simulink model "GolfSwingZVCF"  (R2024a)
settings: Solver=VariableStepAuto  StartTime=0.0  StopTime=StopTime  MaxStep=0.001  RelTol=1e-3
PreLoadFcn:
  | cd(matlabdrive);
PostLoadFcn:
  | %run SCRIPT_mdlWksGenerate.m;
  | mdlWks=get_param('GolfSwingZVCF','ModelWorkspace');
  | mdlWks.DataSource = 'MAT-File';
  | mdlWks.FileName = 'ModelInputs.mat';
  | mdlWks.reload;
model workspace: external: MAT-File ModelInputsZVCF.mat (data not in the file)
undefined symbols (not defined in the file): JointTorqueHip, JointTorqueLElbow, JointTorqueLScap, JointTorqueLShoulder, JointTorqueLWrist, JointTorqueRElbow, JointTorqueRScap, JointTorqueRShoulder, JointTorqueRWrist, JointTorqueTorso, X, Y, Z
libraries: nesl_utility x286, sm_lib x176, matrix_library x11, simulink_extras x2
(part 9 of 9)

== system GolfSwingZVCF/Club/Revolute Joint Shaft Models/12 Segment Shaft (1 Degree Prestress)/ShaftPhysicalConfig/Subsystem8 ==
  Kill : Inport
  KDamp9 : Inport  Port=2
  KShaft9 : Inport  Port=3
  Add : Sum
  Invert : Constant  Value=-1
  Invert1 : Constant  Value=-1
  PS-Simulink Converter11 : nesl_utility/PS-Simulink Converter  PhysicalDomain=network_engine_domain  SubClassName=ps_output  LeftPortType=input  RightPortType=output  PseudoPeriodic=off  Frequencies=[]  VectorFormat=1-D array  Unit=inherit  AffineConversion=off
  PS-Simulink Converter16 : nesl_utility/PS-Simulink Converter  PhysicalDomain=network_engine_domain  SubClassName=ps_output  LeftPortType=input  RightPortType=output  PseudoPeriodic=off  Frequencies=[]  VectorFormat=inherit  Unit=inherit  AffineConversion=off
  Product : Product  Inputs=3
  Product2 : Product
  Product3 : Product  Inputs=3
  Simulink-PS Converter : nesl_utility/Simulink-PS Converter  PhysicalDomain=network_engine_domain  SubClassName=ps_input  LeftPortType=input  RightPortType=output  PseudoPeriodic=off  Frequencies=[]  NoiseDistribution=none  NoiseParameters=[]  Unit=1  AffineConversion=off  FilteringAndDerivatives=provide  SimscapeFilterOrder=1  InputFilterTimeConstant=0.001  UdotUserProvided=0
  Torque9 : PMIOPort  Side=Right
  AV9 : PMIOPort  Port=2  Side=Right
  Position9 : PMIOPort  Port=3  Side=Right
  wires:
  Product3/1 -> Add/1
  Kill/1 -> Product2/1
  KShaft9/1 -> Product/2
  Invert/1 -> Product/3
  Invert1/1 -> Product3/3
  Product/1 -> Add/2
  KDamp9/1 -> Product3/2
  Product2/1 -> Simulink-PS Converter/1
  Add/1 -> Product2/2
  PS-Simulink Converter11/1 -> Product/1
  PS-Simulink Converter16/1 -> Product3/1
  connections:
  Simulink-PS Converter/RConn1 -- Torque9/RConn1
  AV9/RConn1 -- PS-Simulink Converter16/LConn1
  PS-Simulink Converter11/LConn1 -- Position9/RConn1

== system GolfSwingZVCF/Club/Revolute Joint Shaft Models/12 Segment Shaft (1 Degree Prestress)/ShaftPhysicalConfig/Subsystem9 ==
  Kill : Inport
  KDamp10 : Inport  Port=2
  KShaft10 : Inport  Port=3
  Add : Sum
  Invert : Constant  Value=-1
  Invert1 : Constant  Value=-1
  PS-Simulink Converter11 : nesl_utility/PS-Simulink Converter  PhysicalDomain=network_engine_domain  SubClassName=ps_output  LeftPortType=input  RightPortType=output  PseudoPeriodic=off  Frequencies=[]  VectorFormat=1-D array  Unit=inherit  AffineConversion=off
  PS-Simulink Converter16 : nesl_utility/PS-Simulink Converter  PhysicalDomain=network_engine_domain  SubClassName=ps_output  LeftPortType=input  RightPortType=output  PseudoPeriodic=off  Frequencies=[]  VectorFormat=inherit  Unit=inherit  AffineConversion=off
  Product : Product  Inputs=3
  Product2 : Product
  Product3 : Product  Inputs=3
  Simulink-PS Converter : nesl_utility/Simulink-PS Converter  PhysicalDomain=network_engine_domain  SubClassName=ps_input  LeftPortType=input  RightPortType=output  PseudoPeriodic=off  Frequencies=[]  NoiseDistribution=none  NoiseParameters=[]  Unit=1  AffineConversion=off  FilteringAndDerivatives=provide  SimscapeFilterOrder=1  InputFilterTimeConstant=0.001  UdotUserProvided=0
  Torque10 : PMIOPort  Side=Right
  AV10 : PMIOPort  Port=2  Side=Right
  Position10 : PMIOPort  Port=3  Side=Right
  wires:
  Product3/1 -> Add/1
  Kill/1 -> Product2/1
  Invert/1 -> Product/3
  PS-Simulink Converter16/1 -> Product3/1
  Invert1/1 -> Product3/3
  Product/1 -> Add/2
  KDamp10/1 -> Product3/2
  Product2/1 -> Simulink-PS Converter/1
  Add/1 -> Product2/2
  PS-Simulink Converter11/1 -> Product/1
  KShaft10/1 -> Product/2
  connections:
  AV10/RConn1 -- PS-Simulink Converter16/LConn1
  Simulink-PS Converter/RConn1 -- Torque10/RConn1
  PS-Simulink Converter11/LConn1 -- Position10/RConn1

== system GolfSwingZVCF/Club/Revolute Joint Shaft Models/12 Segment Shaft (No Prestress) /ShaftPhysicalConfig/Subsystem ==
  Kill : Inport
  KDamp1 : Inport  Port=2
  KShaft1 : Inport  Port=3
  Add : Sum
  Invert : Constant  Value=-1
  Invert1 : Constant  Value=-1
  PS-Simulink Converter11 : nesl_utility/PS-Simulink Converter  PhysicalDomain=network_engine_domain  SubClassName=ps_output  LeftPortType=input  RightPortType=output  PseudoPeriodic=off  Frequencies=[]  VectorFormat=1-D array  Unit=inherit  AffineConversion=off
  PS-Simulink Converter16 : nesl_utility/PS-Simulink Converter  PhysicalDomain=network_engine_domain  SubClassName=ps_output  LeftPortType=input  RightPortType=output  PseudoPeriodic=off  Frequencies=[]  VectorFormat=inherit  Unit=inherit  AffineConversion=off
  Product : Product  Inputs=3
  Product2 : Product
  Product3 : Product  Inputs=3
  Simulink-PS Converter : nesl_utility/Simulink-PS Converter  PhysicalDomain=network_engine_domain  SubClassName=ps_input  LeftPortType=input  RightPortType=output  PseudoPeriodic=off  Frequencies=[]  NoiseDistribution=none  NoiseParameters=[]  Unit=1  AffineConversion=off  FilteringAndDerivatives=provide  SimscapeFilterOrder=1  InputFilterTimeConstant=0.001  UdotUserProvided=0
  Torque1 : PMIOPort  Side=Right
  AV1 : PMIOPort  Port=2  Side=Right
  Position1 : PMIOPort  Port=3  Side=Right
  wires:
  Product3/1 -> Add/1
  Kill/1 -> Product2/1
  KShaft1/1 -> Product/2
  Invert/1 -> Product/3
  PS-Simulink Converter16/1 -> Product3/1
  Invert1/1 -> Product3/3
  Product/1 -> Add/2
  KDamp1/1 -> Product3/2
  Product2/1 -> Simulink-PS Converter/1
  Add/1 -> Product2/2
  PS-Simulink Converter11/1 -> Product/1
  connections:
  AV1/RConn1 -- PS-Simulink Converter16/LConn1
  Simulink-PS Converter/RConn1 -- Torque1/RConn1
  PS-Simulink Converter11/LConn1 -- Position1/RConn1

== system GolfSwingZVCF/Club/Revolute Joint Shaft Models/12 Segment Shaft (No Prestress) /ShaftPhysicalConfig/Subsystem1 ==
  Kill : Inport
  KDamp2 : Inport  Port=2
  KShaft2 : Inport  Port=3
  Add : Sum
  Invert : Constant  Value=-1
  Invert1 : Constant  Value=-1
  PS-Simulink Converter11 : nesl_utility/PS-Simulink Converter  PhysicalDomain=network_engine_domain  SubClassName=ps_output  LeftPortType=input  RightPortType=output  PseudoPeriodic=off  Frequencies=[]  VectorFormat=1-D array  Unit=inherit  AffineConversion=off
  PS-Simulink Converter16 : nesl_utility/PS-Simulink Converter  PhysicalDomain=network_engine_domain  SubClassName=ps_output  LeftPortType=input  RightPortType=output  PseudoPeriodic=off  Frequencies=[]  VectorFormat=inherit  Unit=inherit  AffineConversion=off
  Product : Product  Inputs=3
  Product2 : Product
  Product3 : Product  Inputs=3
  Simulink-PS Converter : nesl_utility/Simulink-PS Converter  PhysicalDomain=network_engine_domain  SubClassName=ps_input  LeftPortType=input  RightPortType=output  PseudoPeriodic=off  Frequencies=[]  NoiseDistribution=none  NoiseParameters=[]  Unit=1  AffineConversion=off  FilteringAndDerivatives=provide  SimscapeFilterOrder=1  InputFilterTimeConstant=0.001  UdotUserProvided=0
  Torque2 : PMIOPort  Side=Right
  AV2 : PMIOPort  Port=2  Side=Right
  Position2 : PMIOPort  Port=3  Side=Right
  wires:
  Product3/1 -> Add/1
  Kill/1 -> Product2/1
  Invert/1 -> Product/3
  PS-Simulink Converter16/1 -> Product3/1
  Invert1/1 -> Product3/3
  Product/1 -> Add/2
  Product2/1 -> Simulink-PS Converter/1
  Add/1 -> Product2/2
  PS-Simulink Converter11/1 -> Product/1
  KDamp2/1 -> Product3/2
  KShaft2/1 -> Product/2
  connections:
  AV2/RConn1 -- PS-Simulink Converter16/LConn1
  Simulink-PS Converter/RConn1 -- Torque2/RConn1
  PS-Simulink Converter11/LConn1 -- Position2/RConn1

== system GolfSwingZVCF/Club/Revolute Joint Shaft Models/12 Segment Shaft (No Prestress) /ShaftPhysicalConfig/Subsystem10 ==
  Kill : Inport
  KDamp11 : Inport  Port=2
  KShaft11 : Inport  Port=3
  Add : Sum
  Invert : Constant  Value=-1
  Invert1 : Constant  Value=-1
  PS-Simulink Converter11 : nesl_utility/PS-Simulink Converter  PhysicalDomain=network_engine_domain  SubClassName=ps_output  LeftPortType=input  RightPortType=output  PseudoPeriodic=off  Frequencies=[]  VectorFormat=1-D array  Unit=inherit  AffineConversion=off
  PS-Simulink Converter16 : nesl_utility/PS-Simulink Converter  PhysicalDomain=network_engine_domain  SubClassName=ps_output  LeftPortType=input  RightPortType=output  PseudoPeriodic=off  Frequencies=[]  VectorFormat=inherit  Unit=inherit  AffineConversion=off
  Product : Product  Inputs=3
  Product2 : Product
  Product3 : Product  Inputs=3
  Simulink-PS Converter : nesl_utility/Simulink-PS Converter  PhysicalDomain=network_engine_domain  SubClassName=ps_input  LeftPortType=input  RightPortType=output  PseudoPeriodic=off  Frequencies=[]  NoiseDistribution=none  NoiseParameters=[]  Unit=1  AffineConversion=off  FilteringAndDerivatives=provide  SimscapeFilterOrder=1  InputFilterTimeConstant=0.001  UdotUserProvided=0
  Torque11 : PMIOPort  Side=Right
  AV11 : PMIOPort  Port=2  Side=Right
  Position11 : PMIOPort  Port=3  Side=Right
  wires:
  Product3/1 -> Add/1
  Kill/1 -> Product2/1
  Invert/1 -> Product/3
  PS-Simulink Converter16/1 -> Product3/1
  Invert1/1 -> Product3/3
  Product/1 -> Add/2
  Product2/1 -> Simulink-PS Converter/1
  Add/1 -> Product2/2
  PS-Simulink Converter11/1 -> Product/1
  KDamp11/1 -> Product3/2
  KShaft11/1 -> Product/2
  connections:
  AV11/RConn1 -- PS-Simulink Converter16/LConn1
  Simulink-PS Converter/RConn1 -- Torque11/RConn1
  PS-Simulink Converter11/LConn1 -- Position11/RConn1

== system GolfSwingZVCF/Club/Revolute Joint Shaft Models/12 Segment Shaft (No Prestress) /ShaftPhysicalConfig/Subsystem2 ==
  Kill : Inport
  KDamp3 : Inport  Port=2
  KShaft3 : Inport  Port=3
  Add : Sum
  Invert : Constant  Value=-1
  Invert1 : Constant  Value=-1
  PS-Simulink Converter11 : nesl_utility/PS-Simulink Converter  PhysicalDomain=network_engine_domain  SubClassName=ps_output  LeftPortType=input  RightPortType=output  PseudoPeriodic=off  Frequencies=[]  VectorFormat=1-D array  Unit=inherit  AffineConversion=off
  PS-Simulink Converter16 : nesl_utility/PS-Simulink Converter  PhysicalDomain=network_engine_domain  SubClassName=ps_output  LeftPortType=input  RightPortType=output  PseudoPeriodic=off  Frequencies=[]  VectorFormat=inherit  Unit=inherit  AffineConversion=off
  Product : Product  Inputs=3
  Product2 : Product
  Product3 : Product  Inputs=3
  Simulink-PS Converter : nesl_utility/Simulink-PS Converter  PhysicalDomain=network_engine_domain  SubClassName=ps_input  LeftPortType=input  RightPortType=output  PseudoPeriodic=off  Frequencies=[]  NoiseDistribution=none  NoiseParameters=[]  Unit=1  AffineConversion=off  FilteringAndDerivatives=provide  SimscapeFilterOrder=1  InputFilterTimeConstant=0.001  UdotUserProvided=0
  Torque3 : PMIOPort  Side=Right
  AV3 : PMIOPort  Port=2  Side=Right
  Position3 : PMIOPort  Port=3  Side=Right
  wires:
  Product3/1 -> Add/1
  Kill/1 -> Product2/1
  KShaft3/1 -> Product/2
  Invert/1 -> Product/3
  PS-Simulink Converter16/1 -> Product3/1
  Invert1/1 -> Product3/3
  Product/1 -> Add/2
  KDamp3/1 -> Product3/2
  Product2/1 -> Simulink-PS Converter/1
  Add/1 -> Product2/2
  PS-Simulink Converter11/1 -> Product/1
  connections:
  AV3/RConn1 -- PS-Simulink Converter16/LConn1
  Simulink-PS Converter/RConn1 -- Torque3/RConn1
  PS-Simulink Converter11/LConn1 -- Position3/RConn1

== system GolfSwingZVCF/Club/Revolute Joint Shaft Models/12 Segment Shaft (No Prestress) /ShaftPhysicalConfig/Subsystem3 ==
  Kill : Inport
  KDamp4 : Inport  Port=2
  KShaft4 : Inport  Port=3
  Add : Sum
  Invert : Constant  Value=-1
  Invert1 : Constant  Value=-1
  PS-Simulink Converter11 : nesl_utility/PS-Simulink Converter  PhysicalDomain=network_engine_domain  SubClassName=ps_output  LeftPortType=input  RightPortType=output  PseudoPeriodic=off  Frequencies=[]  VectorFormat=1-D array  Unit=inherit  AffineConversion=off
  PS-Simulink Converter16 : nesl_utility/PS-Simulink Converter  PhysicalDomain=network_engine_domain  SubClassName=ps_output  LeftPortType=input  RightPortType=output  PseudoPeriodic=off  Frequencies=[]  VectorFormat=inherit  Unit=inherit  AffineConversion=off
  Product : Product  Inputs=3
  Product2 : Product
  Product3 : Product  Inputs=3
  Simulink-PS Converter : nesl_utility/Simulink-PS Converter  PhysicalDomain=network_engine_domain  SubClassName=ps_input  LeftPortType=input  RightPortType=output  PseudoPeriodic=off  Frequencies=[]  NoiseDistribution=none  NoiseParameters=[]  Unit=1  AffineConversion=off  FilteringAndDerivatives=provide  SimscapeFilterOrder=1  InputFilterTimeConstant=0.001  UdotUserProvided=0
  Torque4 : PMIOPort  Side=Right
  AV4 : PMIOPort  Port=2  Side=Right
  Position4 : PMIOPort  Port=3  Side=Right
  wires:
  Product3/1 -> Add/1
  KShaft4/1 -> Product/2
  Invert/1 -> Product/3
  PS-Simulink Converter16/1 -> Product3/1
  Invert1/1 -> Product3/3
  Product/1 -> Add/2
  KDamp4/1 -> Product3/2
  Product2/1 -> Simulink-PS Converter/1
  Add/1 -> Product2/2
  PS-Simulink Converter11/1 -> Product/1
  Kill/1 -> Product2/1
  connections:
  AV4/RConn1 -- PS-Simulink Converter16/LConn1
  Simulink-PS Converter/RConn1 -- Torque4/RConn1
  PS-Simulink Converter11/LConn1 -- Position4/RConn1

== system GolfSwingZVCF/Club/Revolute Joint Shaft Models/12 Segment Shaft (No Prestress) /ShaftPhysicalConfig/Subsystem4 ==
  Kill : Inport
  KDamp5 : Inport  Port=2
  KShaft5 : Inport  Port=3
  Add : Sum
  Invert : Constant  Value=-1
  Invert1 : Constant  Value=-1
  PS-Simulink Converter11 : nesl_utility/PS-Simulink Converter  PhysicalDomain=network_engine_domain  SubClassName=ps_output  LeftPortType=input  RightPortType=output  PseudoPeriodic=off  Frequencies=[]  VectorFormat=1-D array  Unit=inherit  AffineConversion=off
  PS-Simulink Converter16 : nesl_utility/PS-Simulink Converter  PhysicalDomain=network_engine_domain  SubClassName=ps_output  LeftPortType=input  RightPortType=output  PseudoPeriodic=off  Frequencies=[]  VectorFormat=inherit  Unit=inherit  AffineConversion=off
  Product : Product  Inputs=3
  Product2 : Product
  Product3 : Product  Inputs=3
  Simulink-PS Converter : nesl_utility/Simulink-PS Converter  PhysicalDomain=network_engine_domain  SubClassName=ps_input  LeftPortType=input  RightPortType=output  PseudoPeriodic=off  Frequencies=[]  NoiseDistribution=none  NoiseParameters=[]  Unit=1  AffineConversion=off  FilteringAndDerivatives=provide  SimscapeFilterOrder=1  InputFilterTimeConstant=0.001  UdotUserProvided=0
  Torque5 : PMIOPort  Side=Right
  AV2 : PMIOPort  Port=2  Side=Right
  Position5 : PMIOPort  Port=3  Side=Right
  wires:
  Product3/1 -> Add/1
  KShaft5/1 -> Product/2
  Invert/1 -> Product/3
  PS-Simulink Converter16/1 -> Product3/1
  Invert1/1 -> Product3/3
  Product/1 -> Add/2
  KDamp5/1 -> Product3/2
  Product2/1 -> Simulink-PS Converter/1
  Add/1 -> Product2/2
  PS-Simulink Converter11/1 -> Product/1
  Kill/1 -> Product2/1
  connections:
  AV2/RConn1 -- PS-Simulink Converter16/LConn1
  Simulink-PS Converter/RConn1 -- Torque5/RConn1
  PS-Simulink Converter11/LConn1 -- Position5/RConn1

== system GolfSwingZVCF/Club/Revolute Joint Shaft Models/12 Segment Shaft (No Prestress) /ShaftPhysicalConfig/Subsystem5 ==
  Kill : Inport
  KDamp6 : Inport  Port=2
  KShaft6 : Inport  Port=3
  Add : Sum
  Invert : Constant  Value=-1
  Invert1 : Constant  Value=-1
  PS-Simulink Converter11 : nesl_utility/PS-Simulink Converter  PhysicalDomain=network_engine_domain  SubClassName=ps_output  LeftPortType=input  RightPortType=output  PseudoPeriodic=off  Frequencies=[]  VectorFormat=1-D array  Unit=inherit  AffineConversion=off
  PS-Simulink Converter16 : nesl_utility/PS-Simulink Converter  PhysicalDomain=network_engine_domain  SubClassName=ps_output  LeftPortType=input  RightPortType=output  PseudoPeriodic=off  Frequencies=[]  VectorFormat=inherit  Unit=inherit  AffineConversion=off
  Product : Product  Inputs=3
  Product2 : Product
  Product3 : Product  Inputs=3
  Simulink-PS Converter : nesl_utility/Simulink-PS Converter  PhysicalDomain=network_engine_domain  SubClassName=ps_input  LeftPortType=input  RightPortType=output  PseudoPeriodic=off  Frequencies=[]  NoiseDistribution=none  NoiseParameters=[]  Unit=1  AffineConversion=off  FilteringAndDerivatives=provide  SimscapeFilterOrder=1  InputFilterTimeConstant=0.001  UdotUserProvided=0
  Torque6 : PMIOPort  Side=Right
  AV6 : PMIOPort  Port=2  Side=Right
  Position6 : PMIOPort  Port=3  Side=Right
  wires:
  Product3/1 -> Add/1
  Kill/1 -> Product2/1
  KShaft6/1 -> Product/2
  Invert/1 -> Product/3
  PS-Simulink Converter16/1 -> Product3/1
  Invert1/1 -> Product3/3
  Product/1 -> Add/2
  KDamp6/1 -> Product3/2
  Product2/1 -> Simulink-PS Converter/1
  Add/1 -> Product2/2
  PS-Simulink Converter11/1 -> Product/1
  connections:
  AV6/RConn1 -- PS-Simulink Converter16/LConn1
  Simulink-PS Converter/RConn1 -- Torque6/RConn1
  PS-Simulink Converter11/LConn1 -- Position6/RConn1

== system GolfSwingZVCF/Club/Revolute Joint Shaft Models/12 Segment Shaft (No Prestress) /ShaftPhysicalConfig/Subsystem6 ==
  Kill : Inport
  KDamp7 : Inport  Port=2
  KShaft7 : Inport  Port=3
  Add : Sum
  Invert : Constant  Value=-1
  Invert1 : Constant  Value=-1
  PS-Simulink Converter11 : nesl_utility/PS-Simulink Converter  PhysicalDomain=network_engine_domain  SubClassName=ps_output  LeftPortType=input  RightPortType=output  PseudoPeriodic=off  Frequencies=[]  VectorFormat=1-D array  Unit=inherit  AffineConversion=off
  PS-Simulink Converter16 : nesl_utility/PS-Simulink Converter  PhysicalDomain=network_engine_domain  SubClassName=ps_output  LeftPortType=input  RightPortType=output  PseudoPeriodic=off  Frequencies=[]  VectorFormat=inherit  Unit=inherit  AffineConversion=off
  Product : Product  Inputs=3
  Product2 : Product
  Product3 : Product  Inputs=3
  Simulink-PS Converter : nesl_utility/Simulink-PS Converter  PhysicalDomain=network_engine_domain  SubClassName=ps_input  LeftPortType=input  RightPortType=output  PseudoPeriodic=off  Frequencies=[]  NoiseDistribution=none  NoiseParameters=[]  Unit=1  AffineConversion=off  FilteringAndDerivatives=provide  SimscapeFilterOrder=1  InputFilterTimeConstant=0.001  UdotUserProvided=0
  Torque7 : PMIOPort  Side=Right
  AV7 : PMIOPort  Port=2  Side=Right
  Position7 : PMIOPort  Port=3  Side=Right
  wires:
  Product3/1 -> Add/1
  Kill/1 -> Product2/1
  KShaft7/1 -> Product/2
  Invert/1 -> Product/3
  PS-Simulink Converter16/1 -> Product3/1
  Invert1/1 -> Product3/3
  Product/1 -> Add/2
  KDamp7/1 -> Product3/2
  Product2/1 -> Simulink-PS Converter/1
  Add/1 -> Product2/2
  PS-Simulink Converter11/1 -> Product/1
  connections:
  AV7/RConn1 -- PS-Simulink Converter16/LConn1
  Simulink-PS Converter/RConn1 -- Torque7/RConn1
  PS-Simulink Converter11/LConn1 -- Position7/RConn1

== system GolfSwingZVCF/Club/Revolute Joint Shaft Models/12 Segment Shaft (No Prestress) /ShaftPhysicalConfig/Subsystem7 ==
  Kill : Inport
  KDamp8 : Inport  Port=2
  KShaft8 : Inport  Port=3
  Add : Sum
  Invert : Constant  Value=-1
  Invert1 : Constant  Value=-1
  PS-Simulink Converter11 : nesl_utility/PS-Simulink Converter  PhysicalDomain=network_engine_domain  SubClassName=ps_output  LeftPortType=input  RightPortType=output  PseudoPeriodic=off  Frequencies=[]  VectorFormat=1-D array  Unit=inherit  AffineConversion=off
  PS-Simulink Converter16 : nesl_utility/PS-Simulink Converter  PhysicalDomain=network_engine_domain  SubClassName=ps_output  LeftPortType=input  RightPortType=output  PseudoPeriodic=off  Frequencies=[]  VectorFormat=inherit  Unit=inherit  AffineConversion=off
  Product : Product  Inputs=3
  Product2 : Product
  Product3 : Product  Inputs=3
  Simulink-PS Converter : nesl_utility/Simulink-PS Converter  PhysicalDomain=network_engine_domain  SubClassName=ps_input  LeftPortType=input  RightPortType=output  PseudoPeriodic=off  Frequencies=[]  NoiseDistribution=none  NoiseParameters=[]  Unit=1  AffineConversion=off  FilteringAndDerivatives=provide  SimscapeFilterOrder=1  InputFilterTimeConstant=0.001  UdotUserProvided=0
  Torque8 : PMIOPort  Side=Right
  AV8 : PMIOPort  Port=2  Side=Right
  Position8 : PMIOPort  Port=3  Side=Right
  wires:
  Product3/1 -> Add/1
  Kill/1 -> Product2/1
  KShaft8/1 -> Product/2
  Invert/1 -> Product/3
  PS-Simulink Converter16/1 -> Product3/1
  Invert1/1 -> Product3/3
  Product/1 -> Add/2
  Product2/1 -> Simulink-PS Converter/1
  Add/1 -> Product2/2
  PS-Simulink Converter11/1 -> Product/1
  KDamp8/1 -> Product3/2
  connections:
  AV8/RConn1 -- PS-Simulink Converter16/LConn1
  Simulink-PS Converter/RConn1 -- Torque8/RConn1
  PS-Simulink Converter11/LConn1 -- Position8/RConn1

== system GolfSwingZVCF/Club/Revolute Joint Shaft Models/12 Segment Shaft (No Prestress) /ShaftPhysicalConfig/Subsystem8 ==
  Kill : Inport
  KDamp9 : Inport  Port=2
  KShaft9 : Inport  Port=3
  Add : Sum
  Invert : Constant  Value=-1
  Invert1 : Constant  Value=-1
  PS-Simulink Converter11 : nesl_utility/PS-Simulink Converter  PhysicalDomain=network_engine_domain  SubClassName=ps_output  LeftPortType=input  RightPortType=output  PseudoPeriodic=off  Frequencies=[]  VectorFormat=1-D array  Unit=inherit  AffineConversion=off
  PS-Simulink Converter16 : nesl_utility/PS-Simulink Converter  PhysicalDomain=network_engine_domain  SubClassName=ps_output  LeftPortType=input  RightPortType=output  PseudoPeriodic=off  Frequencies=[]  VectorFormat=inherit  Unit=inherit  AffineConversion=off
  Product : Product  Inputs=3
  Product2 : Product
  Product3 : Product  Inputs=3
  Simulink-PS Converter : nesl_utility/Simulink-PS Converter  PhysicalDomain=network_engine_domain  SubClassName=ps_input  LeftPortType=input  RightPortType=output  PseudoPeriodic=off  Frequencies=[]  NoiseDistribution=none  NoiseParameters=[]  Unit=1  AffineConversion=off  FilteringAndDerivatives=provide  SimscapeFilterOrder=1  InputFilterTimeConstant=0.001  UdotUserProvided=0
  Torque9 : PMIOPort  Side=Right
  AV9 : PMIOPort  Port=2  Side=Right
  Position9 : PMIOPort  Port=3  Side=Right
  wires:
  Product3/1 -> Add/1
  Kill/1 -> Product2/1
  KShaft9/1 -> Product/2
  Invert/1 -> Product/3
  Invert1/1 -> Product3/3
  Product/1 -> Add/2
  KDamp9/1 -> Product3/2
  Product2/1 -> Simulink-PS Converter/1
  Add/1 -> Product2/2
  PS-Simulink Converter11/1 -> Product/1
  PS-Simulink Converter16/1 -> Product3/1
  connections:
  Simulink-PS Converter/RConn1 -- Torque9/RConn1
  AV9/RConn1 -- PS-Simulink Converter16/LConn1
  PS-Simulink Converter11/LConn1 -- Position9/RConn1

== system GolfSwingZVCF/Club/Revolute Joint Shaft Models/12 Segment Shaft (No Prestress) /ShaftPhysicalConfig/Subsystem9 ==
  Kill : Inport
  KDamp10 : Inport  Port=2
  KShaft10 : Inport  Port=3
  Add : Sum
  Invert : Constant  Value=-1
  Invert1 : Constant  Value=-1
  PS-Simulink Converter11 : nesl_utility/PS-Simulink Converter  PhysicalDomain=network_engine_domain  SubClassName=ps_output  LeftPortType=input  RightPortType=output  PseudoPeriodic=off  Frequencies=[]  VectorFormat=1-D array  Unit=inherit  AffineConversion=off
  PS-Simulink Converter16 : nesl_utility/PS-Simulink Converter  PhysicalDomain=network_engine_domain  SubClassName=ps_output  LeftPortType=input  RightPortType=output  PseudoPeriodic=off  Frequencies=[]  VectorFormat=inherit  Unit=inherit  AffineConversion=off
  Product : Product  Inputs=3
  Product2 : Product
  Product3 : Product  Inputs=3
  Simulink-PS Converter : nesl_utility/Simulink-PS Converter  PhysicalDomain=network_engine_domain  SubClassName=ps_input  LeftPortType=input  RightPortType=output  PseudoPeriodic=off  Frequencies=[]  NoiseDistribution=none  NoiseParameters=[]  Unit=1  AffineConversion=off  FilteringAndDerivatives=provide  SimscapeFilterOrder=1  InputFilterTimeConstant=0.001  UdotUserProvided=0
  Torque10 : PMIOPort  Side=Right
  AV10 : PMIOPort  Port=2  Side=Right
  Position10 : PMIOPort  Port=3  Side=Right
  wires:
  Product3/1 -> Add/1
  Kill/1 -> Product2/1
  Invert/1 -> Product/3
  PS-Simulink Converter16/1 -> Product3/1
  Invert1/1 -> Product3/3
  Product/1 -> Add/2
  KDamp10/1 -> Product3/2
  Product2/1 -> Simulink-PS Converter/1
  Add/1 -> Product2/2
  PS-Simulink Converter11/1 -> Product/1
  KShaft10/1 -> Product/2
  connections:
  AV10/RConn1 -- PS-Simulink Converter16/LConn1
  Simulink-PS Converter/RConn1 -- Torque10/RConn1
  PS-Simulink Converter11/LConn1 -- Position10/RConn1

== matlab function GolfSwingZVCF/Club/Impact Model/Golf Ball Reaction Force ==
  data: u input; FImpact output
function FImpact = fcn(u)

FImpact=-u*1.5*.44704*.0459/.0005;
%Impact Time = 0.0005 s
%Golf Ball Mass = 0.0459 g
%MPH to m/s conversion = 0.44704 m/s / MPH
%Smash Factor = 1.5

== matlab function GolfSwingZVCF/Club/Clubhead Air Resistance Calculator/Drag Function ==
  data: u input; FDrag output
function FDrag = fcn(u)

FDrag = -1/2*1.225*3.1415927*(2.5/39)^2*0.47*u^2;
%Shape Factor = 0.47
%Air Density = 1.225 kg/m3
%CH Radius = 2.5"
%Fd=-1/2*Density*ShapeFactor*CSA*v^2

== matlab function GolfSwingZVCF/RJM Inputs/Hip Input Torque ==
  data: JointTorqueHipsInput input; JointTorqueHips output
function JointTorqueHips = fcn(JointTorqueHipsInput)
JointTorqueHips=JointTorqueHipsInput;

== matlab function GolfSwingZVCF/RJM Inputs/Torso Input Torque ==
  data: JointTorqueTorsoInput input; JointTorqueHips output
function JointTorqueHips = fcn(JointTorqueTorsoInput)
JointTorqueHips=JointTorqueTorsoInput;

== matlab function GolfSwingZVCF/RJM Inputs/LScap Input Torque ==
  data: JointTorqueHipsInput input; JointTorqueHips output
function JointTorqueHips = fcn(JointTorqueHipsInput)
JointTorqueHips=JointTorqueHipsInput;

== matlab function GolfSwingZVCF/RJM Inputs/RScap Input Torque ==
  data: JointTorqueRScapInput input; JointTorqueRScap output
function JointTorqueRScap = fcn(JointTorqueRScapInput)
JointTorqueRScap=JointTorqueRScapInput;

== matlab function GolfSwingZVCF/RJM Inputs/LShoulder Input Torque ==
  data: JointTorqueLShoulderInput input; JointTorqueLShoulder output
function JointTorqueLShoulder = fcn(JointTorqueLShoulderInput)
JointTorqueLShoulder=JointTorqueLShoulderInput;

== matlab function GolfSwingZVCF/RJM Inputs/LWrist Input Torque ==
  data: JointTorqueLWristInput input; JointTorqueLWrist output
function JointTorqueLWrist = fcn(JointTorqueLWristInput)
JointTorqueLWrist=JointTorqueLWristInput;

== matlab function GolfSwingZVCF/RJM Inputs/RShoulder Input Torque ==
  data: JointTorqueRShoulderInput input; JointTorqueRShoulder output
function JointTorqueRShoulder = fcn(JointTorqueRShoulderInput)
JointTorqueRShoulder=JointTorqueRShoulderInput;

== matlab function GolfSwingZVCF/RJM Inputs/RWrist Input Torque ==
  data: JointTorqueRWristInput input; JointTorqueRWrist output
function JointTorqueRWrist = fcn(JointTorqueRWristInput)
JointTorqueRWrist=JointTorqueRWristInput;

== matlab function GolfSwingZVCF/RJM Inputs/Left Elbow Input Torque ==
  data: JointTorqueLElbowInput input; JointTorqueLElbow output
function JointTorqueLElbow = fcn(JointTorqueLElbowInput)
JointTorqueLElbow=JointTorqueLElbowInput;

== matlab function GolfSwingZVCF/RJM Inputs/Right Elbow Input Torque ==
  data: JointTorqueRElbowInput input; JointTorqueRElbow output
function JointTorqueRElbow = fcn(JointTorqueRElbowInput)
JointTorqueRElbow=JointTorqueRElbowInput;

== matlab function GolfSwingZVCF/Club/CHGlobal/Filtering Block/MATLAB Function ==
  data: u input; y output
function y = fcn(u)
% Need to figure out how to design a filter and use the filtfilt function
% as it is a zero phase shift filter.

% function y = fcn(u)
% 
% y = filtfilt();
